simulink model "feedback_linearization"  (R2024a)
settings: Solver=VariableStepAuto  StartTime=0.0  StopTime=15  RelTol=1e-3
settings Model: Creator=PC  LastModifiedBy=PC
settings SolverCC: MaxConsecutiveMinStep=10

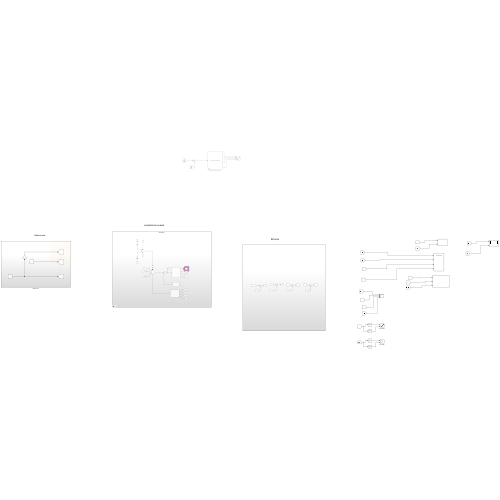
[thumbnail: Simulink's stored preview of the top-level diagram]
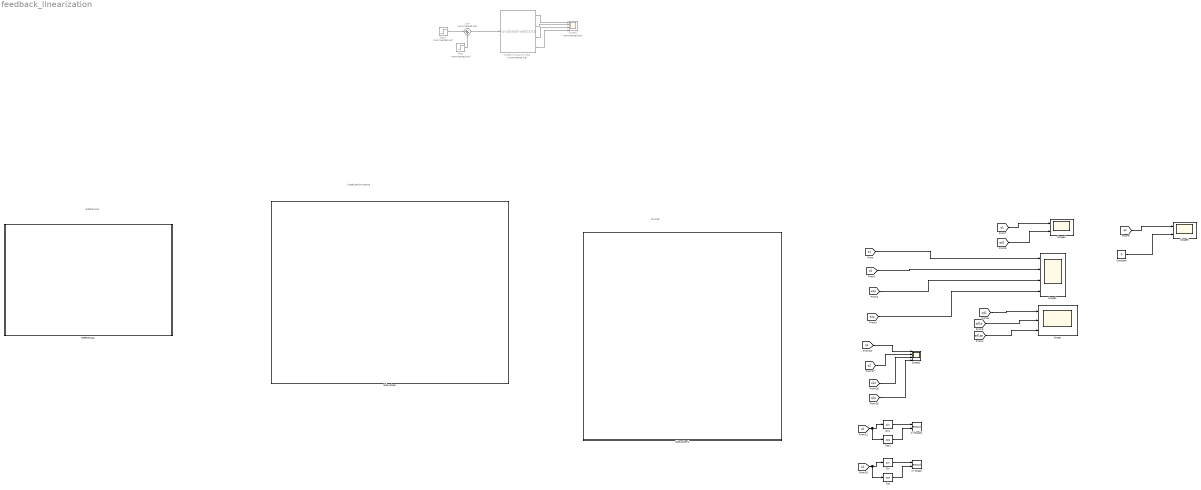
== system feedback_linearization ==
  note: Errores
  note: Linealización exacta
  note: Referencias
  Constant : Constant  Value=0
  Cos : Trigonometry  Operator=cos
  Cos1 : Trigonometry  Operator=cos
  Modelo Furuta No-lineal : M-S-Function  Commented=on  FunctionName=FurutanolinealSLV2  Parameters=parameter1,parameter2,parameter3,parameter4  mask{parameter1=0, parameter2=0, parameter3=0, parameter4=0}
      mask prompts: parameter1 "Phi(q1)"; parameter2 "Theta(q2)"; parameter3 "dPhi(q1p)"; parameter4 "dTheta(q2p)"
  Referencias : Subsystem
  Scope : Scope  NumInputPorts=3
  Scope1 : Scope  NumInputPorts=4
  Scope2 : Scope  NumInputPorts=4
  Scope3 : Scope  Commented=on  NumInputPorts=4
  Scope4 : Scope  NumInputPorts=2
  Scope5 : Scope  NumInputPorts=2
  Sin : Trigonometry
  Sin1 : Trigonometry
  Step : Step  Commented=on  Time=0.5  SampleTime=0
  Step1 : Step  Commented=on  After=-1  SampleTime=0
  Subsystem : Subsystem  Variant=on  VariantControlMode=label  VariantControl=Subsystem  LabelModeActiveChoice=Subsystem
  Subsystem1 : Subsystem
  Sum : Sum  Commented=on  Inputs=|++
  XY Graph : Record  FileSettingsInternal="{\"entries\":[{\"content\":{\"excelSettings\":{\"content\":{},\"type\":\"Streamout.ExcelSettings\"}},\"type\":\"Streamout.FileSettingStorage\",\"uuid\":\"\"}],\"packageUris\":[\"http:\\/\\/schema.mathworks.com\\/mf0\\/streamout_blocks\\/R2020a\"],\"version\":\"1.0\"}"  Layout=[1 1]  SignalsInternal="{\"entries\":[{\"content\":{\"signals\":[{\"content\":{\"blockPath\":[],\"dimensions\":[1],\"domain\":\"\",\"lineColor\":\"#a2142f\",\"plots\":[ 1 ],\"port\":1,\"sid\":[\"\"],\"signalID\":1,\"signalName\":\"Sin\"},\"type\":\"RecordBlkView.Signal\",\"uuid\":\"\"},{\"content\":{\"blockPath\":[],\"dimensions\":[1],\"domain\":\"\",\"lineColor\":\"#139fff\",\"plots\":[ 1 ],\"port\":2,\"sid\":[\"\"],\"signalID\":2,\"signalName\":\"Cos\"},\"type\":\"RecordBlkView.Signal\",\"uuid\":\"\"}]},\"type\":\"RecordBlkView.InputSignals\",\"uuid\":\"\"}],\"packageUris\":[\"http:\\/\\/schema.mathworks.com\\/mf0\\/streamout_blocks\\/R2020a\"],\"version\":\"1.0\"}"  VisualizationBindings="{\"xyplotplugin\":{\"info\":[{\"series\":[{\"bindingParametersList\":[{\"parameter\":\"X-Axis\",\"signalID\":1,\"signalName\":\"Sin\"},{\"parameter\":\"Y-Axis\",\"signalID\":2,\"signalName\":\"Cos\"}],\"seriesID\":0}],\"subplotID\":1}]}}"  CompatibilityTag=XY
  XY Graph1 : Record  FileSettingsInternal="{\"entries\":[{\"content\":{\"excelSettings\":{\"content\":{},\"type\":\"Streamout.ExcelSettings\"}},\"type\":\"Streamout.FileSettingStorage\",\"uuid\":\"\"}],\"packageUris\":[\"http:\\/\\/schema.mathworks.com\\/mf0\\/streamout_blocks\\/R2020a\"],\"version\":\"1.0\"}"  Layout=[1 1]  SignalsInternal="{\"entries\":[{\"content\":{\"signals\":[{\"content\":{\"blockPath\":[],\"dimensions\":[1],\"domain\":\"\",\"lineColor\":\"#a2142f\",\"plots\":[ 1 ],\"port\":1,\"sid\":[\"\"],\"signalID\":1,\"signalName\":\"Sin1\"},\"type\":\"RecordBlkView.Signal\",\"uuid\":\"\"},{\"content\":{\"blockPath\":[],\"dimensions\":[1],\"domain\":\"\",\"lineColor\":\"#139fff\",\"plots\":[ 1 ],\"port\":2,\"sid\":[\"\"],\"signalID\":2,\"signalName\":\"Cos1\"},\"type\":\"RecordBlkView.Signal\",\"uuid\":\"\"}]},\"type\":\"RecordBlkView.InputSignals\",\"uuid\":\"\"}],\"packageUris\":[\"http:\\/\\/schema.mathworks.com\\/mf0\\/streamout_blocks\\/R2020a\"],\"version\":\"1.0\"}"  VisualizationBindings="{\"xyplotplugin\":{\"info\":[{\"series\":[{\"bindingParametersList\":[{\"parameter\":\"X-Axis\",\"signalID\":1,\"signalName\":\"Sin1\"},{\"parameter\":\"Y-Axis\",\"signalID\":2,\"signalName\":\"Cos1\"}],\"seriesID\":0}],\"subplotID\":1}]}}"  CompatibilityTag=XY
  wires:
  [q1p] -> Scope1/3
  [q1] -> Scope1/1
  [q2] -> Scope1/2
  [q2p] -> Scope1/4
  Sin1/1 -> XY Graph1/1
  [q1] -> Cos/1, Sin/1
  Cos1/1 -> XY Graph1/2
  Cos/1 -> XY Graph/2
  Sin/1 -> XY Graph/1
  [q2] -> Cos1/1, Sin1/1
  [e2] -> Scope2/2
  [e1p] -> Scope2/3
  [e2p] -> Scope2/4
  [e1] -> Scope2/1
  [qd1] -> Scope/1
  [qd1p] -> Scope/2
  [qd1pp] -> Scope/3
  Modelo Furuta No-lineal/1 -> Scope3/1
  Modelo Furuta No-lineal/2 -> Scope3/2
  Modelo Furuta No-lineal/3 -> Scope3/3
  Modelo Furuta No-lineal/4 -> Scope3/4
  Sum/1 -> Modelo Furuta No-lineal/1
  Step/1 -> Sum/2
  Step1/1 -> Sum/1
  [q1] -> Scope4/1
  [qd1] -> Scope4/2
  [q2] -> Scope5/1
  Constant/1 -> Scope5/2

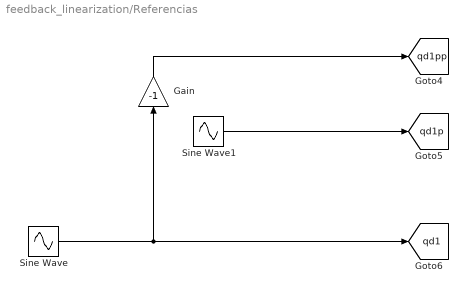
== system feedback_linearization/Referencias ==
  Gain : Gain  Gain=-1
  Sine Wave : Sin  SampleTime=0
  Sine Wave1 : Sin  Phase=90  SampleTime=0
  tag scope: qd1=global, qd1p=global, qd1pp=global
  wires:
  Gain/1 -> [qd1pp]
  Sine Wave/1 -> Gain/1, [qd1]
  Sine Wave1/1 -> [qd1p]

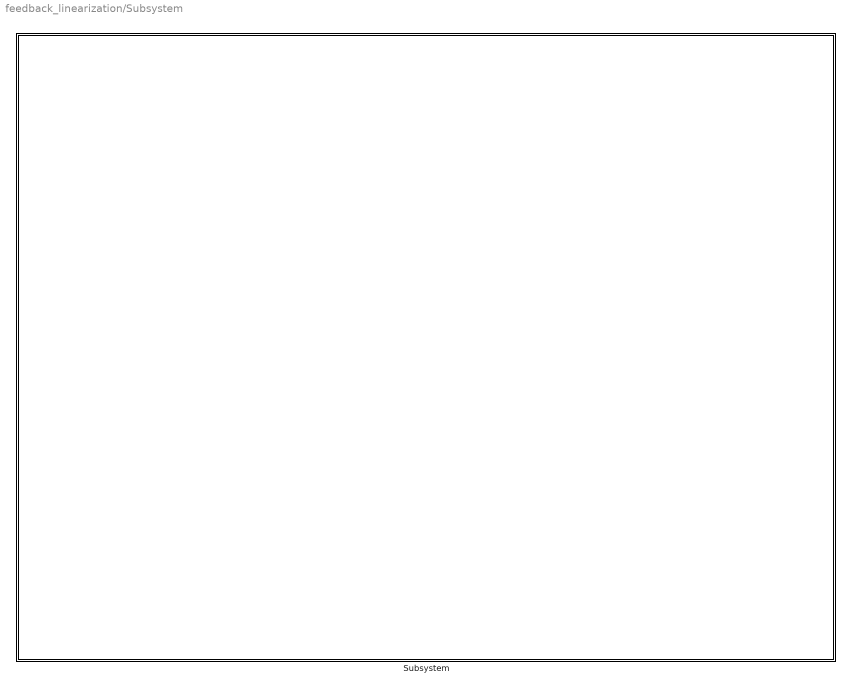
== system feedback_linearization/Subsystem ==
  Subsystem : Subsystem  VariantControl=Subsystem

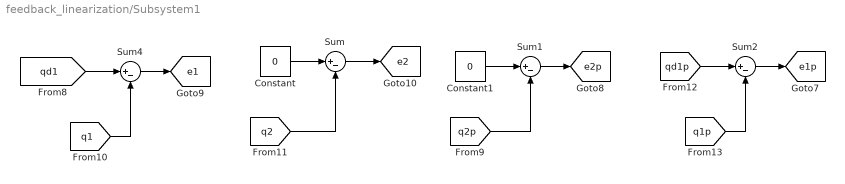
== system feedback_linearization/Subsystem1 ==
  Constant : Constant  Value=0
  Constant1 : Constant  Value=0
  Sum{,1..2,4} (4 alike) : Sum  Inputs=|+-
  tag scope: e1=global, e1p=global, e2=global, e2p=global
  wires:
  [q1] -> Sum4/2
  [qd1p] -> Sum2/1
  [q1p] -> Sum2/2
  Sum4/1 -> [e1]
  Sum/1 -> [e2]
  [qd1] -> Sum4/1
  Sum2/1 -> [e1p]
  Constant/1 -> Sum/1
  [q2] -> Sum/2
  Constant1/1 -> Sum1/1
  [q2p] -> Sum1/2
  Sum1/1 -> [e2p]

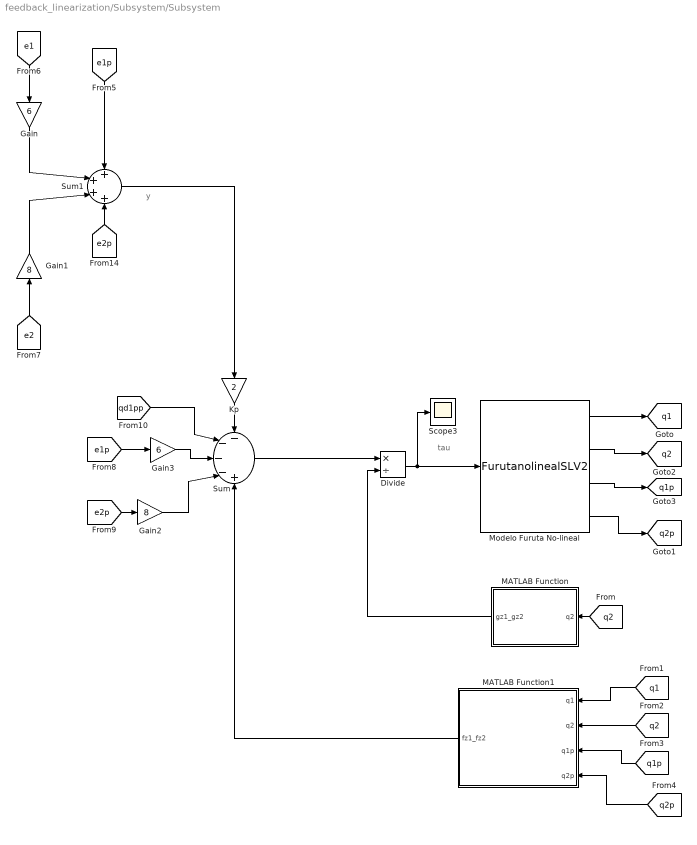
== system feedback_linearization/Subsystem/Subsystem ==
  note: y
  note: tau
  Divide : Product  Inputs=*/
  Gain : Gain  Gain=6
  Gain1 : Gain  Gain=8
  Gain2 : Gain  Gain=8
  Gain3 : Gain  Gain=6
  Kp : Gain  Gain=2
  MATLAB Function : MATLAB Function  TreatAsAtomicUnit=on
  MATLAB Function1 : MATLAB Function  TreatAsAtomicUnit=on
  Modelo Furuta No-lineal : M-S-Function  FunctionName=FurutanolinealSLV2  Parameters=parameter1,parameter2,parameter3,parameter4  mask{parameter1=0, parameter2=0, parameter3=0, parameter4=0}
      mask prompts: parameter1 "Phi(q1)"; parameter2 "Theta(q2)"; parameter3 "dPhi(q1p)"; parameter4 "dTheta(q2p)"
  Scope3 : Scope
  Sum : Sum  Inputs=----+
  Sum1 : Sum  Inputs=++++
  tag scope: q1=global, q1p=global, q2=global, q2p=global
  wires:
  [q2] -> MATLAB Function/1(q2)
  Divide/1 -> Scope3/1, Modelo Furuta No-lineal/1
  [q1p] -> MATLAB Function1/3(q1p)
  [e2p] -> Sum1/4
  Modelo Furuta No-lineal/3 -> [q1p]
  MATLAB Function/1(gz1_gz2) -> Divide/2
  Modelo Furuta No-lineal/2 -> [q2]
  Modelo Furuta No-lineal/4 -> [q2p]
  [e1p] -> Sum1/1
  [e2] -> Gain1/1
  Gain/1 -> Sum1/2
  [q1] -> MATLAB Function1/1(q1)
  [q2] -> MATLAB Function1/2(q2)
  [q2p] -> MATLAB Function1/4(q2p)
  [e1] -> Gain/1
  Gain1/1 -> Sum1/3
  Modelo Furuta No-lineal/1 -> [q1]
  Sum/1 -> Divide/1
  Kp/1 -> Sum/1
  Sum1/1 -> Kp/1
  MATLAB Function1/1(fz1_fz2) -> Sum/5
  [e2p] -> Gain2/1
  [e1p] -> Gain3/1
  Gain3/1 -> Sum/3
  Gain2/1 -> Sum/4
  [qd1pp] -> Sum/2

== matlab function feedback_linearization/Subsystem/Subsystem/MATLAB Function1 ==
  data: q1 input; q2 input; fz1_fz2 output; q1p input; q2p input
function fz1_fz2  = fz_sum(q1,q2,q1p,q2p)
 betha = 100;
  tetha1 =  0.0619;
  tetha2 =  0.0149;
  tetha3 =  0.0185;
  tetha4 =  0.0131;
  tetha5 =  0.5076;
  tetha6 =  0.0083;
  tetha7 =  0.0007;
  tetha8 =  0.0188;
  tetha9 =  0.0087;
  
  M11 = tetha1 + tetha2*sin(q2)^2;
  M12 = tetha3*cos(q2);
  M21 = M12;
  M22 = tetha4;

  M = [M11 M12;M21 M22];

  C11 = 0.5*tetha2*q2p*sin(2*q2);
  C12 = -tetha3*q2p*sin(q2) + 0.5*tetha2*q1*sin(2*q2);
  C21 = -0.5*tetha2*q1p*sin(2*q2);
  C22 = 0;

  C = [C11 C12;C21 C22];
  g1 = 0;
  g2 = -tetha5*sin(q2);

  g = [g1;g2];

  fv1 = tetha6*q1p;
  fv2 = tetha7*q2p;

  fv = [fv1;fv2];

  fc1 = tetha8*tanh(betha*q1p);
  fc2 = tetha9*tanh(betha*q2p);
  
  fc = [fc1;fc2];

  Qp = [q1p;q2p];
  
  fz = M\(-C*Qp-g-fv-fc);

  fz1_fz2 = fz(1)+fz(2);

end

== matlab function feedback_linearization/Subsystem/Subsystem/MATLAB Function ==
  data: q2 input; gz1_gz2 output
function gz1_gz2  = gz_div(q2)
      tetha1 =  0.0619;
  tetha2 =  0.0149;
  tetha3 =  0.0185;
  tetha4 =  0.0131;
  tetha5 =  0.5076;
  tetha6 =  0.0083;
  tetha7 =  0.0007;
  tetha8 =  0.0188;
  tetha9 =  0.0087;


    M11 = tetha1 + tetha2*sin(q2)^2;
  M12 = tetha3*cos(q2);
  M21 = M12;
  M22 = tetha4;

  M = [M11 M12;M21 M22];

   
        gz = (1/det(M))*[M22 ;-M12];
   gz1_gz2 = -1*(gz(1)+gz(2));
end
